simulink model "finalprojectnonlinsim"  (R2025b)
settings: Solver=VariableStepAuto  StartTime=0.0  StopTime=20  FixedStep=0.003  RelTol=1e-3
values from neighbouring files (symbols this model uses):
  K = lqr(A, B, Q, R)    [FinalProject.m]
settings Model: Creator=alexi  LastModifiedBy=alexi
settings DataIOCC: ReturnWorkspaceOutputs=off

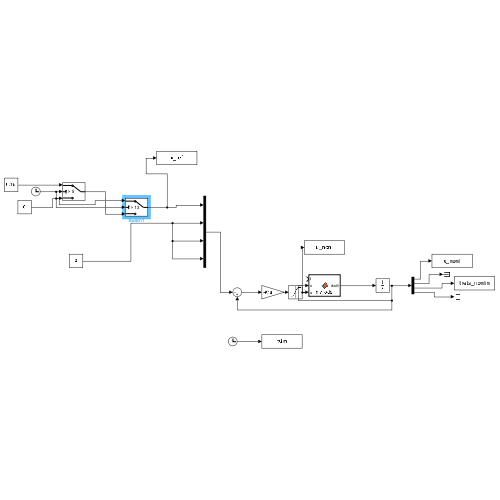
[thumbnail: Simulink's stored preview of the top-level diagram]
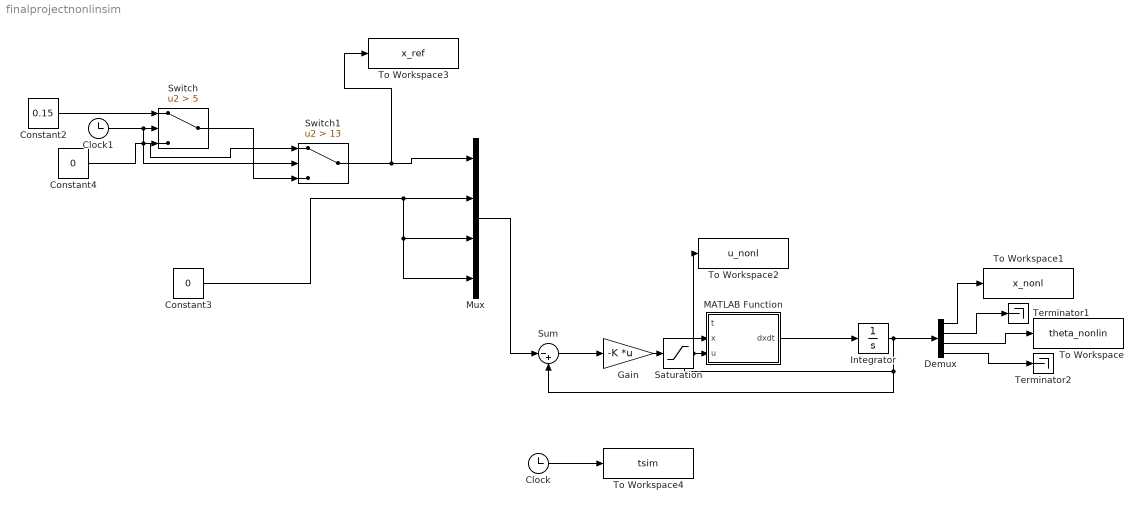
== system finalprojectnonlinsim ==
  Clock : Clock
  Clock1 : Clock
  Constant2 : Constant  Value=0.15
  Constant3 : Constant  Value=0
  Constant4 : Constant  Value=0
  Demux : Demux
  Gain : Gain  Gain=-K  Multiplication=Matrix(K*u)
  Integrator : Integrator  InitialCondition=[0;0;0;0]
  MATLAB Function : MATLAB Function  TreatAsAtomicUnit=on
  Mux : Mux
  Saturation : Saturate  UpperLimit=9  LowerLimit=-9
  Sum : Sum  Inputs=|-+
  Switch : Switch  Criteria=u2 > Threshold  Threshold=5  SaturateOnIntegerOverflow=off  InputSameDT=off
  Switch1 : Switch  Criteria=u2 > Threshold  Threshold=13  SaturateOnIntegerOverflow=off  InputSameDT=off
  Terminator1 : Terminator
  Terminator2 : Terminator
  To Workspace : ToWorkspace  VariableName=theta_nonlin  SampleTime=-1
      settings: Save2DSignal=2-D array (concatenate along first dimension)
  To Workspace1 : ToWorkspace  VariableName=x_nonl  SampleTime=-1
      settings: Save2DSignal=2-D array (concatenate along first dimension)
  To Workspace2 : ToWorkspace  VariableName=u_nonl  SampleTime=-1
      settings: Save2DSignal=2-D array (concatenate along first dimension)
  To Workspace3 : ToWorkspace  VariableName=x_ref  SampleTime=-1
      settings: Save2DSignal=2-D array (concatenate along first dimension)
  To Workspace4 : ToWorkspace  VariableName=tsim  SampleTime=-1
      settings: Save2DSignal=2-D array (concatenate along first dimension)
  wires:
  Sum/1 -> Gain/1
  Mux/1 -> Sum/1
  MATLAB Function/1(dxdt) -> Integrator/1
  Clock/1 -> To Workspace4/1
  Demux/3 -> To Workspace/1
  Integrator/1 -> Sum/2, MATLAB Function/2(x), Demux/1
  Demux/1 -> To Workspace1/1
  Demux/2 -> Terminator1/1
  Demux/4 -> Terminator2/1
  Saturation/1 -> To Workspace2/1, MATLAB Function/3(u)
  Gain/1 -> Saturation/1
  Constant3/1 -> Mux/2, Mux/4, Mux/3
  Switch1/1 -> To Workspace3/1, Mux/1
  Constant4/1 -> Switch1/1, Switch/3
  Switch/1 -> Switch1/3
  Clock1/1 -> Switch1/2, Switch/2
  Constant2/1 -> Switch/1

== matlab function finalprojectnonlinsim/MATLAB Function ==
  data: t input; x input; u input; dxdt output
function dxdt = my_ode(t, x, u)
    Rm = 13;
    Kb = 0.155;
    Kt = 0.1;
    Rw = 0.022;
    
    dx1 = x(2);  
    dx2 = (72057594037927936*(3104590330245044102605*sin(x(3))*x(4)^2 + 49084432098735875140000000*((Kt/Rm)*(u-Kb*(-x(2)/Rw-x(4)))) - 205668190026137654525952*cos(x(3))*sin(x(3)) + 7292228516638307123200000*((Kt/Rm)*(u-Kb*(-x(2)/Rw-x(4))))*cos(x(3))))/(5*(302139754198141619704189581397317386240*cos(x(3))^2 - 2583356202112353832612568201949451968449));
    dx3 = x(4);
    dx4 = (36028797018963968*(41930313970670265958400*cos(x(3))*sin(x(3))*x(4)^2 + 842093866964841039965600000*((Kt/Rm)*(u-Kb*(-x(2)/Rw-x(4)))) - 23750204900409635480929791*sin(x(3)) + 662929865148937011200000000*((Kt/Rm)*(u-Kb*(-x(2)/Rw-x(4))))*cos(x(3))))/(5*(302139754198141619704189581397317386240*cos(x(3))^2 - 2583356202112353832612568201949451968449));

    dxdt = [dx1; dx2; dx3; dx4];
end
